simulink model "anode"  (R2018b)
settings: Solver=VariableStepAuto  StartTime=0.0  StopTime=1000  RelTol=1e-3
settings Model: Creator=10537  LastModifiedBy=10537

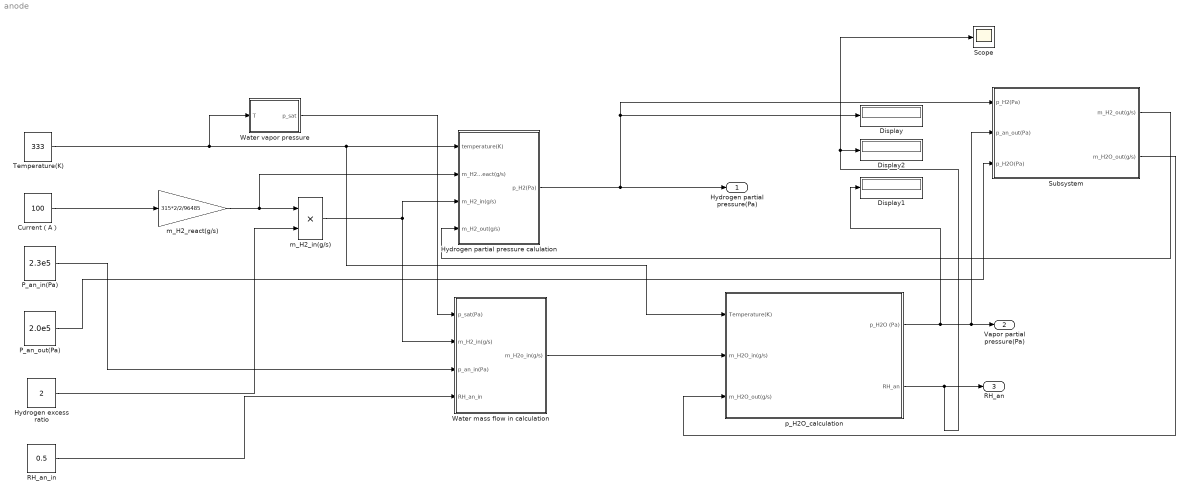
== system anode ==
  "Current（A） " : Constant  Value=100
  Display : Display
  Display1 : Display
  Display2 : Display
  "Hydrogen excess ratio " : Constant  Value=2
  Hydrogen partial pressure calulation : Subsystem
  "P_an_in(Pa) " : Constant  Value=2.3e5
  "P_an_out(Pa) " : Constant  Value=2.0e5
  RH_an_in : Constant  Value=0.5
  Scope : Scope
  Subsystem : Subsystem
  Temperature(K) : Constant  Value=333
  Water mass flow in calculation : Subsystem
  Water vapor pressure : MATLAB Function  TreatAsAtomicUnit=on
  m_H2_in(g/s) : Product
  m_H2_react(g/s) : Gain  Gain=315*2/2/96485
  p_H2O_calculation : Subsystem
  "Hydrogen partial pressure(Pa) " : Outport
  Vapor partial pressure(Pa) : Outport  Port=2
  "RH_an " : Outport  Port=3
  wires:
  "Current（A） "/1 -> m_H2_react(g/s)/1
  m_H2_react(g/s)/1 -> Hydrogen partial pressure calulation/2(m_H2_react(g/s)), m_H2_in(g/s)/1
  Temperature(K)/1 -> Water vapor pressure/1(T), p_H2O_calculation/1(Temperature(K)), Hydrogen partial pressure calulation/1(temperature(K))
  m_H2_in(g/s)/1 -> Water mass flow in calculation/2(m_H2_in(g/s)), Hydrogen partial pressure calulation/3(m_H2_in(g/s))
  Hydrogen partial pressure calulation/1(p_H2(Pa)) -> Display/1, Subsystem/1(p_H2(Pa)), "Hydrogen partial pressure(Pa) "/1
  "Hydrogen excess ratio "/1 -> m_H2_in(g/s)/2
  Water vapor pressure/1(p_sat) -> Water mass flow in calculation/1(p_sat(Pa))
  "P_an_in(Pa) "/1 -> Water mass flow in calculation/3(p_an_in(Pa))
  RH_an_in/1 -> Water mass flow in calculation/4(RH_an_in)
  Water mass flow in calculation/1(m_H2o_in(g/s)) -> p_H2O_calculation/2(m_H2O_in(g/s))
  p_H2O_calculation/1(p_H2O (Pa)) -> Display1/1, Subsystem/2(p_an_out(Pa)), Vapor partial pressure(Pa)/1
  p_H2O_calculation/2("RH_an ") -> Scope/1, Display2/1, "RH_an "/1
  "P_an_out(Pa) "/1 -> Subsystem/3(p_H2O(Pa))
  Subsystem/1(m_H2_out(g/s)) -> Hydrogen partial pressure calulation/4(m_H2_out(g/s))
  Subsystem/2(m_H2O_out(g/s)) -> p_H2O_calculation/3(m_H2O_out(g/s))

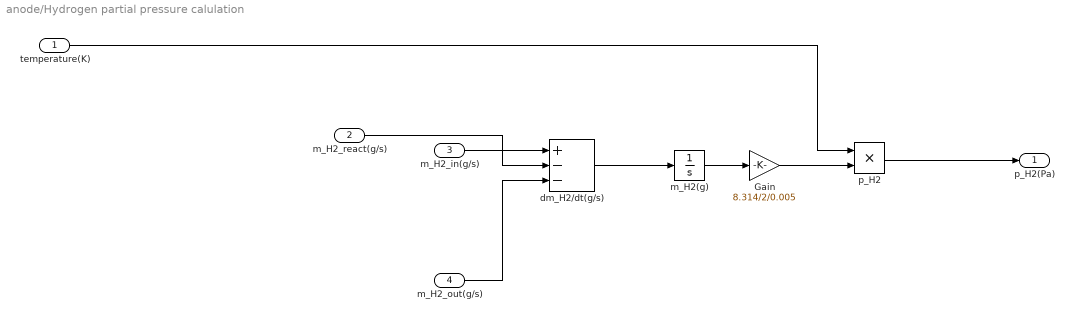
== system anode/Hydrogen partial pressure calulation ==
  temperature(K) : Inport
  m_H2_react(g/s) : Inport  Port=2
  m_H2_in(g/s) : Inport  Port=3
  m_H2_out(g/s) : Inport  Port=4
  Gain : Gain  Gain=8.314/2/0.005
  dm_H2/dt(g/s) : Sum  Inputs=+--
  m_H2(g) : Integrator  InitialCondition=0.01
  p_H2 : Product
  p_H2(Pa) : Outport
  wires:
  m_H2_in(g/s)/1 -> dm_H2/dt(g/s)/1
  m_H2(g)/1 -> Gain/1
  m_H2_react(g/s)/1 -> dm_H2/dt(g/s)/2
  Gain/1 -> p_H2/2
  dm_H2/dt(g/s)/1 -> m_H2(g)/1
  p_H2/1 -> p_H2(Pa)/1
  m_H2_out(g/s)/1 -> dm_H2/dt(g/s)/3
  temperature(K)/1 -> p_H2/1

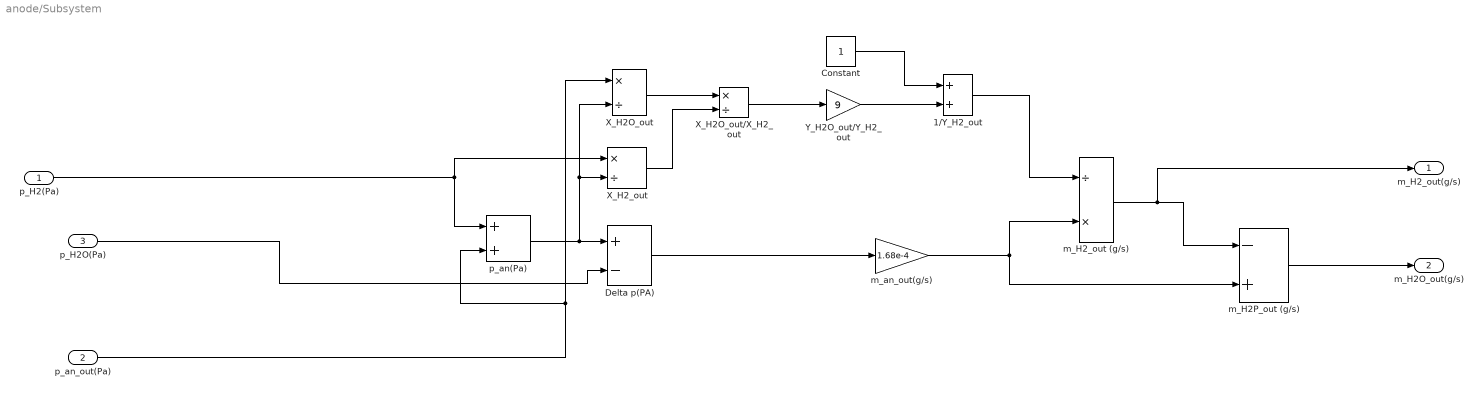
== system anode/Subsystem ==
  p_H2(Pa) : Inport
  p_an_out(Pa) : Inport  Port=2
  p_H2O(Pa) : Inport  Port=3
  1/Y_H2_out : Sum
  Constant : Constant
  Delta p(PA) : Sum  Inputs=+-
  X_H2O_out : Product  Inputs=*/
  X_H2O_out/X_H2_out : Product  Inputs=*/
  X_H2_out : Product  Inputs=*/
  Y_H2O_out/Y_H2_out : Gain  Gain=9
  m_H2P_out (g/s) : Sum  Inputs=-+
  m_H2_out (g/s) : Product  Inputs=/*
  m_an_out(g/s) : Gain  Gain=1.68e-4
  p_an(Pa) : Sum
  m_H2_out(g/s) : Outport
  m_H2O_out(g/s) : Outport  Port=2
  wires:
  Delta p(PA)/1 -> m_an_out(g/s)/1
  X_H2O_out/X_H2_out/1 -> Y_H2O_out/Y_H2_out/1
  p_an(Pa)/1 -> X_H2_out/2, X_H2O_out/2, Delta p(PA)/1
  p_H2(Pa)/1 -> p_an(Pa)/1, X_H2_out/1
  m_H2_out (g/s)/1 -> m_H2_out(g/s)/1, m_H2P_out (g/s)/1
  m_an_out(g/s)/1 -> m_H2P_out (g/s)/2, m_H2_out (g/s)/2
  1/Y_H2_out/1 -> m_H2_out (g/s)/1
  p_an_out(Pa)/1 -> p_an(Pa)/2, X_H2O_out/1
  Y_H2O_out/Y_H2_out/1 -> 1/Y_H2_out/2
  Constant/1 -> 1/Y_H2_out/1
  X_H2_out/1 -> X_H2O_out/X_H2_out/2
  X_H2O_out/1 -> X_H2O_out/X_H2_out/1
  m_H2P_out (g/s)/1 -> m_H2O_out(g/s)/1
  p_H2O(Pa)/1 -> Delta p(PA)/2

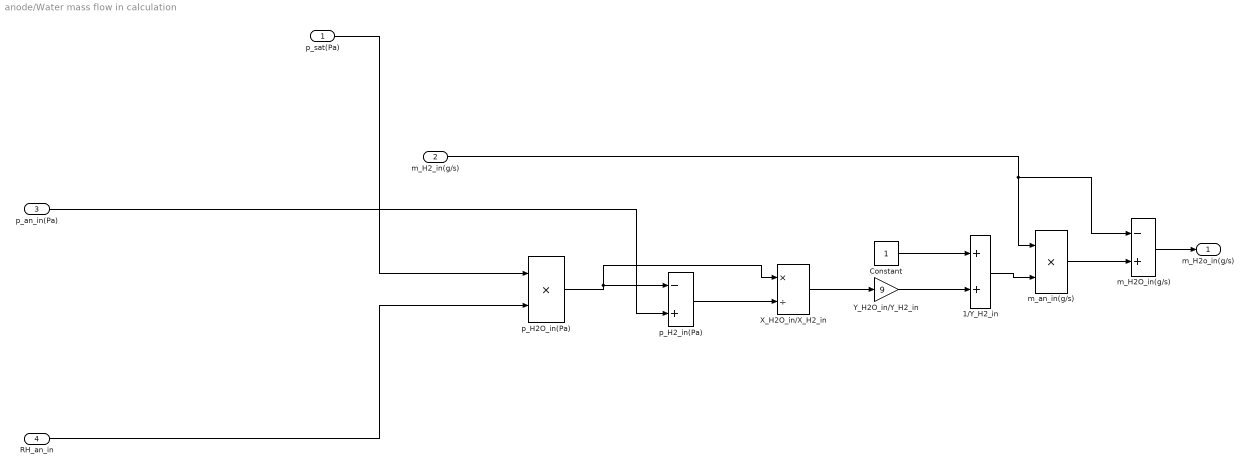
== system anode/Water mass flow in calculation ==
  p_sat(Pa) : Inport
  m_H2_in(g/s) : Inport  Port=2
  p_an_in(Pa) : Inport  Port=3
  RH_an_in : Inport  Port=4
  1/Y_H2_in : Sum
  Constant : Constant
  X_H2O_in/X_H2_in : Product  Inputs=*/
  Y_H2O_in/Y_H2_in : Gain  Gain=9
  m_H2O_in(g/s) : Sum  Inputs=-+
  m_an_in(g/s) : Product
  p_H2O_in(Pa) : Product
  p_H2_in(Pa) : Sum  Inputs=-+
  m_H2o_in(g/s) : Outport
  wires:
  1/Y_H2_in/1 -> m_an_in(g/s)/2
  m_an_in(g/s)/1 -> m_H2O_in(g/s)/2
  m_H2_in(g/s)/1 -> m_an_in(g/s)/1, m_H2O_in(g/s)/1
  p_an_in(Pa)/1 -> p_H2_in(Pa)/2
  Y_H2O_in/Y_H2_in/1 -> 1/Y_H2_in/2
  X_H2O_in/X_H2_in/1 -> Y_H2O_in/Y_H2_in/1
  Constant/1 -> 1/Y_H2_in/1
  p_H2_in(Pa)/1 -> X_H2O_in/X_H2_in/2
  p_H2O_in(Pa)/1 -> X_H2O_in/X_H2_in/1, p_H2_in(Pa)/1
  m_H2O_in(g/s)/1 -> m_H2o_in(g/s)/1
  p_sat(Pa)/1 -> p_H2O_in(Pa)/1
  RH_an_in/1 -> p_H2O_in(Pa)/2

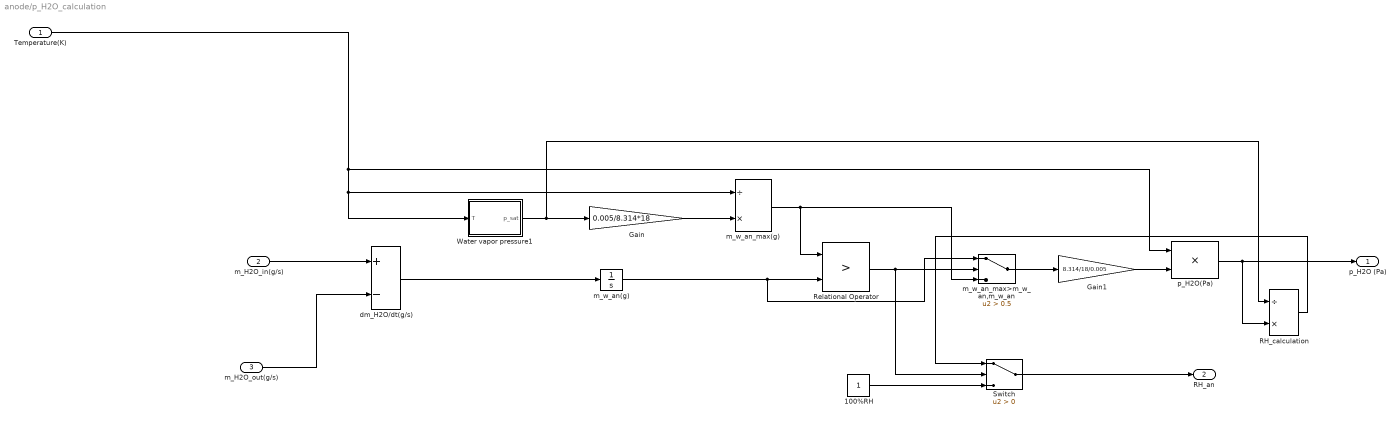
== system anode/p_H2O_calculation ==
  Temperature(K) : Inport
  m_H2O_in(g/s) : Inport  Port=2
  m_H2O_out(g/s) : Inport  Port=3
  100%RH : Constant
  Gain : Gain  Gain=0.005/8.314*18
  Gain1 : Gain  Gain=8.314/18/0.005
  "RH_calculation " : Product  Inputs=/*
  Relational Operator : RelationalOperator  Operator=>  OutDataTypeStr=boolean  RndMeth=Simplest
  Switch : Switch  Criteria=u2 > Threshold
  Water vapor pressure1 : MATLAB Function  TreatAsAtomicUnit=on
  dm_H2O/dt(g/s) : Sum  Inputs=+-
  m_w_an(g) : Integrator  InitialCondition=0.01
  m_w_an_max(g) : Product  Inputs=/*
  m_w_an_max>m_w_an,m_w_an : Switch  Criteria=u2 > Threshold  Threshold=0.5
  p_H2O(Pa) : Product
  p_H2O (Pa) : Outport
  "RH_an " : Outport  Port=2
  wires:
  Temperature(K)/1 -> Water vapor pressure1/1(T), m_w_an_max(g)/1, p_H2O(Pa)/1
  100%RH/1 -> Switch/3
  m_w_an_max(g)/1 -> m_w_an_max>m_w_an,m_w_an/3, Relational Operator/1
  dm_H2O/dt(g/s)/1 -> m_w_an(g)/1
  Switch/1 -> "RH_an "/1
  m_w_an(g)/1 -> m_w_an_max>m_w_an,m_w_an/1, Relational Operator/2
  Water vapor pressure1/1(p_sat) -> "RH_calculation "/1, Gain/1
  Relational Operator/1 -> Switch/2, m_w_an_max>m_w_an,m_w_an/2
  p_H2O(Pa)/1 -> p_H2O (Pa)/1, "RH_calculation "/2
  Gain1/1 -> p_H2O(Pa)/2
  m_w_an_max>m_w_an,m_w_an/1 -> Gain1/1
  "RH_calculation "/1 -> Switch/1
  Gain/1 -> m_w_an_max(g)/2
  m_H2O_out(g/s)/1 -> dm_H2O/dt(g/s)/2
  m_H2O_in(g/s)/1 -> dm_H2O/dt(g/s)/1

== matlab function anode/p_H2O_calculation/Water vapor pressure1 ==
  data: T input; p_sat output
function p_sat = fcn(T)%%求水的分压，饱和蒸汽压

p_sat = exp(23.196-3816.44/(T-46.13));

== matlab function anode/Water vapor pressure ==
  data: T input; p_sat output
function p_sat = fcn(T)%%求水的分压，饱和蒸汽压

p_sat = exp(23.196-3816.44/(T-46.13));
